simulink model "Factory"  (R2022b)
settings: Solver=VariableStepAuto  StartTime=0.0  StopTime=10.0  RelTol=1e-3
settings Model: Creator=Stefano  LastModifiedBy=stefanopanzieri
settings SolverCC: AlgebraicLoopSolver=TrustRegion
settings DebuggingCC: UnconnectedInputMsg=warning  UnconnectedOutputMsg=warning  UnconnectedLineMsg=warning  SFMachineParentedDataDiag=warning
settings ModelReferenceCC: EnableRefExpFcnMdlSchedulingChecks=on
settings SFSimCC: CustomCodeUndefinedFunction=UseInterfaceOnly
settings RTWCC: DLArmComputeVersion=19.05

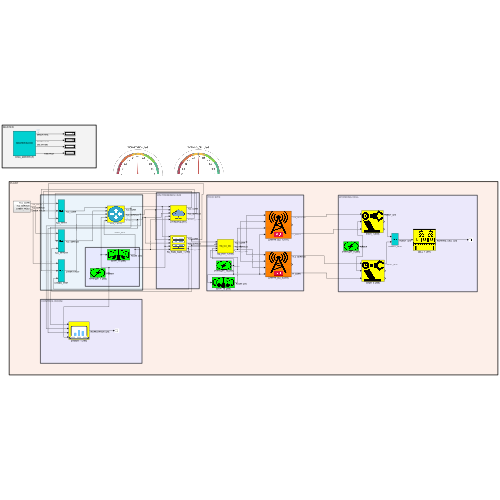
[thumbnail: Simulink's stored preview of the top-level diagram]
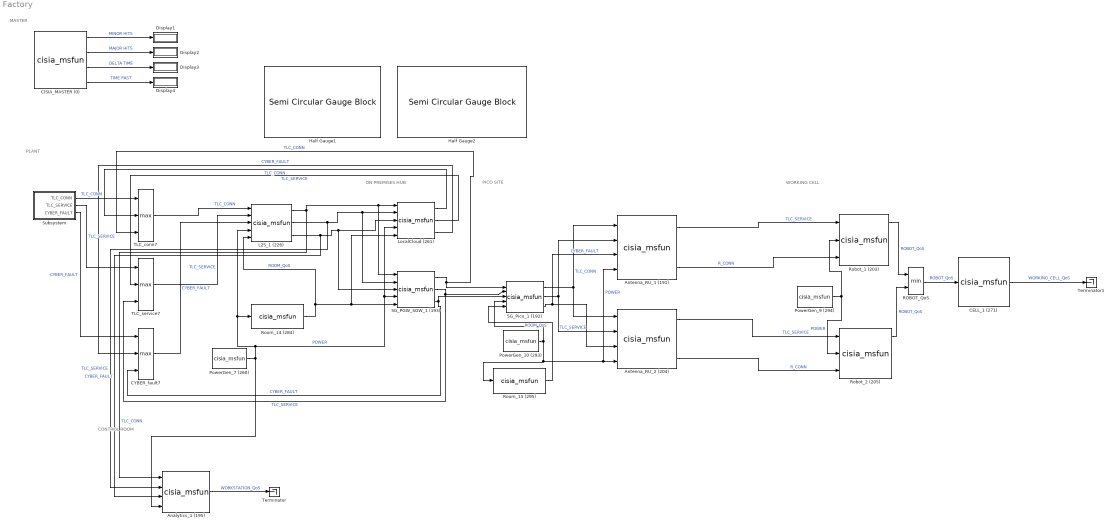
== system Factory ==
  note: WORKING CELL
  note: PICO SITE
  note: CONTROL ROOM
  note: ON PREMISES HUB
  note: PLANT
  note: MASTER
  5G_PGW_SGW_1 (193) : M-S-Function  FunctionName=cisia_msfun  Parameters=Parameter1, Parameter2, Parameter3, resources, Parameter10, codeupdate, step_received, step_computed, dynamic_computed, step_sended, id_entity, id_project, id_type, name_type, color  mask(S-function:msfcn_unit_delay){Parameter1='5G_PGW_SGW_1', Parameter2=1, Parameter3='ORO', resources=|, Parameter10=off, codeupdate=off, step_received=|, step_computed=, dynamic_computed=, step_sended=|, id_entity=193, id_project=34, id_type=40, name_type=App_Server, color=#00AAFF}
      mask resources=|
      | *** INPUT RESOURCES ***
      | NUM_INPUTS 5
      | TLC_CONN (20)
      | TLC_SERVICE (20)
      | CYBER_FAULT (10)
      | POWER (1)
      | ROOM_QoS (1)
      |
      | *** STATE VARIABLES ***
      | NUM_VARIABLES 24
      | Operative_Level(NUMERIC)(1)(1)
      | TLC_services(NUMERIC_ARRAY)(20)(0  0  0  0  0  0  0  0  0  0  0  0  0  0  0  0  0  0  0  0)
      | TLC_service_names(STRING)(100)()
      | Connection(NUMERIC_ARRAY)(20)(0  0  0  0  0  0  0  0  0  0  0  0  0  0  0  0  0  0  0  0)
      | Dos_attack(NUMERIC)(1)(0)
      | MITM_attack(NUMERIC)(1)(0)
      | Virus_Attack(NUMERIC)(1)(0)
      | Port_Scan_Attack(NUMERIC)(1)(0)
      | Cyber_Fault(NUMERIC_ARRAY)(10)(0  0  0  0  0  0  0  0  0  0)
      | BGP_hijacking(NUMERIC)(1)(0)
      | Mechanical_Fault(NUMERIC)(1)(0)
      | Cooling_Fault(NUMERIC)(1)(0)
      | Conn_Fault(NUMERIC)(1)(0)
      | Consumed_Services(NUMERIC_ARRAY)(20)(0  0  0  0  0  0  0  0  0  0  0  0  0  0  0  0  0  0  0  0)
      | Service_Fault(NUMERIC)(1)(0)
      | Redundancy_Fault(NUMERIC)(1)(0)
      | BotNet_Attack(NUMERIC)(1)(0)
      | Data_Corruption(NUMERIC)(1)(0)
      | syslog_adm_login(NUMERIC)(1)(0)
      | SW_Change(NUMERIC)(1)(0)
      | Config_Change(NUMERIC)(1)(0)
      | Port_Saturation(NUMERIC)(1)(0)
      | Congestion_Fault(NUMERIC)(1)(0)
      | TLC_revoke(NUMERIC_ARRAY)(20)(0  0  0  0  0  0  0  0  0  0  0  0  0  0  0  0  0  0  0  0)
      |
      | *** OUTPUT RESOURCES ***
      | NUM_OUTPUTS 3
      | TLC_CONN (20)
      | TLC_SERVICE (20)
      | CYBER_FAULT (10)
      mask step_received=|
      | Connection=max(Connection_init,TLC_CONN);
      | TLC_services=max(TLC_services_init,TLC_SERVICE);
      | TLC_services=mod(TLC_services,10);
      | TLC_revoke=floor(TLC_SERVICE/10);
      |
      | Mechanical_Fault=max([Mechanical_Fault Mechanical_Fault_init]);
      |
      | %if strcmp(name_entity,"BlockChainServer") && (cisia.major_time>=2)
      |  % Dos_attack=1;
      |  %TLC_revoke(9)=1;
      |  %TLC_services(9)=0;
      | %end
      |
      |
      | Cyber_Fault=max(CYBER_FAULT, transpose([Dos_attack   MITM_attack Virus_Attack Port_Scan_Attack  BGP_hijacking BotNet_Attack Data_Corruption SW_Change Config_Change Port_Saturation]));
      |
      | Service_Fault=max(abs(Consumed_Services.*TLC_services-Consumed_Services));
      | Redundancy_Fault=max(abs(Consumed_Services.*TLC_CONN-Consumed_Services));
      |
      | Conn_Fault=max([Dos_attack  Mechanical_Fault  1-POWER 1-ROOM_QoS] );
      |
      |
      | Operative_Level=(1-Conn_Fault)*(1-0.5*max(Cyber_Fault))*(1-Service_Fault)*max(max(TLC_CONN),0.5);
      mask step_sended=|
      | TLC_CONN=Connection*(1-Conn_Fault);
      | TLC_SERVICE=TLC_services*(1-Conn_Fault)*(1-Service_Fault)*(1-syslog_adm_login)+10*TLC_revoke;
      | CYBER_FAULT=Cyber_Fault*(1-Conn_Fault);
      mask prompts: Parameter1 "entity name"; Parameter2 "sampling time"; Parameter3 "project"; resources "input resources and state variables"; Parameter10 "Bring state variables to output"; codeupdate "update code from mask"
      mask help: This is a level-2 MATLAB file S-function which demonstrates CISIA entity
      mask DialogControl Container1 Prompt: All parameters
      mask Display: image('Icons/App_Server.png')
  5G_Pico_1 (192) : M-S-Function  FunctionName=cisia_msfun  Parameters=Parameter1, Parameter2, Parameter3, resources, Parameter10, codeupdate, step_received, step_computed, dynamic_computed, step_sended, id_entity, id_project, id_type, name_type, color  mask(S-function:msfcn_unit_delay){Parameter1='5G_Pico_1', Parameter2=1, Parameter3='ORO', resources=|, Parameter10=off, codeupdate=off, step_received=|, step_computed=, dynamic_computed=, step_sended=|, id_entity=192, id_project=34, id_type=42, name_type=5G_CU_DU, color=#FF00FF}
      mask resources=|
      | *** INPUT RESOURCES ***
      | NUM_INPUTS 5
      | TLC_CONN (20)
      | TLC_SERVICE (20)
      | CYBER_FAULT (10)
      | POWER (1)
      | ROOM_QoS (1)
      |
      | *** STATE VARIABLES ***
      | NUM_VARIABLES 20
      | Operative_Level(NUMERIC)(1)(1)
      | TLC_services(NUMERIC_ARRAY)(20)(0  0  0  0  0  0  0  0  0  0  0  0  0  0  0  0  0  0  0  0)
      | Connection(NUMERIC_ARRAY)(20)(0  0  0  0  0  0  0  0  0  0  0  0  0  0  0  0  0  0  0  0)
      | Dos_attack(NUMERIC)(1)(0)
      | MITM_attack(NUMERIC)(1)(0)
      | Virus_Attack(NUMERIC)(1)(0)
      | Port_Scan_Attack(NUMERIC)(1)(0)
      | Cyber_Fault(NUMERIC_ARRAY)(10)(0  0  0  0  0  0  0  0  0  0)
      | BGP_hijacking(NUMERIC)(1)(0)
      | Mechanical_Fault(NUMERIC)(1)(0)
      | Conn_Fault(NUMERIC)(1)(0)
      | Consumed_Services(NUMERIC_ARRAY)(20)(0  0  0  0  0  0  0  0  0  0  0  0  0  0  0  0  0  0  0  0)
      | Service_Fault(NUMERIC)(1)(0)
      | Redundancy_Fault(NUMERIC)(1)(0)
      | BotNet_Attack(NUMERIC)(1)(0)
      | Data_Corruption(NUMERIC)(1)(0)
      | SW_Change(NUMERIC)(1)(0)
      | Config_Change(NUMERIC)(1)(0)
      | Port_Saturation(NUMERIC)(1)(0)
      | TLC_revoke(NUMERIC_ARRAY)(20)(0  0  0  0  0  0  0  0  0  0  0  0  0  0  0  0  0  0  0  0)
      |
      | *** OUTPUT RESOURCES ***
      | NUM_OUTPUTS 3
      | TLC_CONN (20)
      | TLC_SERVICE (20)
      | CYBER_FAULT (10)
      mask step_received=|
      | Connection=max(Connection_init,TLC_CONN);
      | TLC_services=max(TLC_services_init,TLC_SERVICE);
      | TLC_services=mod(TLC_services,10);
      | TLC_revoke=floor(TLC_SERVICE/10);
      |
      | Cyber_Fault=max(CYBER_FAULT, transpose([Dos_attack   MITM_attack Virus_Attack Port_Scan_Attack  BGP_hijacking BotNet_Attack Data_Corruption SW_Change Config_Change Port_Saturation]));
      |
      | Conn_Fault=max([Dos_attack  Mechanical_Fault  1-POWER 1-ROOM_QoS] );
      |
      | Service_Fault=max(abs(Consumed_Services.*TLC_services-Consumed_Services));
      | Redundancy_Fault=max(abs(Consumed_Services.*TLC_CONN-Consumed_Services));
      |
      | Operative_Level=(1-Conn_Fault)*(1-0.5*max(Cyber_Fault))*(1-Service_Fault)*max(max(TLC_CONN),0.5);
      mask step_sended=|
      | TLC_CONN=Connection*(1-Conn_Fault);
      | TLC_SERVICE=TLC_services*(1-Conn_Fault)*(1-Service_Fault)+TLC_revoke*10;
      | CYBER_FAULT=Cyber_Fault*(1-Conn_Fault);
      mask prompts: Parameter1 "entity name"; Parameter2 "sampling time"; Parameter3 "project"; resources "input resources and state variables"; Parameter10 "Bring state variables to output"; codeupdate "update code from mask"
      mask help: This is a level-2 MATLAB file S-function which demonstrates CISIA entity
      mask DialogControl Container1 Prompt: All parameters
      mask Display: disp('5G_CU_DU')
  Analytics_1 (195) : M-S-Function  FunctionName=cisia_msfun  Parameters=Parameter1, Parameter2, Parameter3, resources, Parameter10, codeupdate, step_received, step_computed, dynamic_computed, step_sended, id_entity, id_project, id_type, name_type, color  mask(S-function:msfcn_unit_delay){Parameter1='Analytics_1', Parameter2=1, Parameter3='ORO', resources=|, Parameter10=off, codeupdate=off, step_received=|, step_computed=, dynamic_computed=, step_sended=WORKSTATION_QoS=Operative_Level;, id_entity=195, id_project=34, id_type=43, name_type=Workstation, color=#FFFFFF}
      mask resources=|
      | *** INPUT RESOURCES ***
      | NUM_INPUTS 4
      | TLC_CONN (20)
      | TLC_SERVICE (20)
      | CYBER_FAULT (10)
      | POWER (1)
      |
      | *** STATE VARIABLES ***
      | NUM_VARIABLES 18
      | Operative_Level(NUMERIC)(1)(1)
      | Connection(NUMERIC_ARRAY)(20)(0  0  0  0  0  0  0  0  0  0  0  0  0  0  0  0  0  0  0  0)
      | Dos_attack(NUMERIC)(1)(0)
      | MITM_attack(NUMERIC)(1)(0)
      | Virus_Attack(NUMERIC)(1)(0)
      | Port_Scan_Attack(NUMERIC)(1)(0)
      | Cyber_Fault(NUMERIC_ARRAY)(10)(0  0  0  0  0  0  0  0  0  0)
      | BGP_hijacking(NUMERIC)(1)(0)
      | Mechanical_Fault(NUMERIC)(1)(0)
      | Conn_Fault(NUMERIC)(1)(0)
      | Consumed_Services(NUMERIC_ARRAY)(20)(0  0  0  0  0  0  0  0  0  0  0  0  0  0  0  0  0  0  0  0)
      | Service_Fault(NUMERIC)(1)(0)
      | Redundancy_Fault(NUMERIC)(1)(0)
      | BotNet_Attack(NUMERIC)(1)(0)
      | Data_Corruption(NUMERIC)(1)(0)
      | SW_Change(NUMERIC)(1)(0)
      | Config_Change(NUMERIC)(1)(0)
      | Port_Saturation(NUMERIC)(1)(0)
      |
      | *** OUTPUT RESOURCES ***
      | NUM_OUTPUTS 1
      | WORKSTATION_QoS (1)
      mask step_received=|
      | Connection=max(Connection_init,TLC_CONN);
      |
      | Cyber_Fault=max(CYBER_FAULT, transpose([Dos_attack   MITM_attack Virus_Attack Port_Scan_Attack  BGP_hijacking BotNet_Attack Data_Corruption SW_Change Config_Change Port_Saturation]));
      |
      | % Vale 1 in presenza di fault
      | Conn_Fault=max([Dos_attack  Mechanical_Fault  1-POWER] );
      |
      |
      |
      | Operative_Level=(1-Conn_Fault)*max(max(TLC_CONN),0.5);
      mask prompts: Parameter1 "entity name"; Parameter2 "sampling time"; Parameter3 "project"; resources "input resources and state variables"; Parameter10 "Bring state variables to output"; codeupdate "update code from mask"
      mask help: This is a level-2 MATLAB file S-function which demonstrates CISIA entity
      mask DialogControl Container1 Prompt: All parameters
      mask Display: image('Icons/Analytics_1.png')
  Antenna_RU_1 (191) : M-S-Function  FunctionName=cisia_msfun  Parameters=Parameter1, Parameter2, Parameter3, resources, Parameter10, codeupdate, step_received, step_computed, dynamic_computed, step_sended, id_entity, id_project, id_type, name_type, color  mask(S-function:msfcn_unit_delay){Parameter1='Antenna_RU_1', Parameter2=1, Parameter3='ORO', resources=|, Parameter10=off, codeupdate=off, step_received=|, step_computed=, dynamic_computed=, step_sended=|, id_entity=191, id_project=34, id_type=41, name_type=RU_ANTENNA, color=#FFFFFF}
      mask resources=|
      | *** INPUT RESOURCES ***
      | NUM_INPUTS 4
      | TLC_CONN (20)
      | TLC_SERVICE (20)
      | CYBER_FAULT (10)
      | POWER (1)
      |
      | *** STATE VARIABLES ***
      | NUM_VARIABLES 24
      | Operative_Level(NUMERIC)(1)(1)
      | TLC_services(NUMERIC_ARRAY)(20)(0  0  0  0  0  0  0  0  0  0  0  0  0  0  0  0  0  0  0  0)
      | TLC_service_names(STRING)(100)()
      | Connection(NUMERIC_ARRAY)(20)(0  0  0  0  0  0  0  0  0  0  0  0  0  0  0  0  0  0  0  0)
      | Dos_attack(NUMERIC)(1)(0)
      | MITM_attack(NUMERIC)(1)(0)
      | Virus_Attack(NUMERIC)(1)(0)
      | Port_Scan_Attack(NUMERIC)(1)(0)
      | Cyber_Fault(NUMERIC_ARRAY)(10)(0  0  0  0  0  0  0  0  0  0)
      | BGP_hijacking(NUMERIC)(1)(0)
      | Mechanical_Fault(NUMERIC)(1)(0)
      | Power_Fault(NUMERIC)(1)(0)
      | Conn_Fault(NUMERIC)(1)(0)
      | Consumed_Services(NUMERIC_ARRAY)(20)(0  0  0  0  0  0  0  0  0  0  0  0  0  0  0  0  0  0  0  0)
      | Service_Fault(NUMERIC)(1)(0)
      | Redundancy_Fault(NUMERIC)(1)(0)
      | BotNet_Attack(NUMERIC)(1)(0)
      | Data_Corruption(NUMERIC)(1)(0)
      | SW_Change(NUMERIC)(1)(0)
      | Config_Change(NUMERIC)(1)(0)
      | Port_Saturation(NUMERIC)(1)(0)
      | Congestion_Fault(NUMERIC)(1)(0)
      | My_Service(NUMERIC)(1)(0)
      | TLC_revoke(NUMERIC_ARRAY)(20)(0  0  0  0  0  0  0  0  0  0  0  0  0  0  0  0  0  0  0  0)
      |
      | *** OUTPUT RESOURCES ***
      | NUM_OUTPUTS 3
      | TLC_SERVICE (20)
      | CYBER_FAULT (10)
      | R_CONN (20)
      mask step_received=|
      | Connection=max(Connection_init,TLC_CONN);
      | TLC_services=max(TLC_services_init,TLC_SERVICE);
      | TLC_services=mod(TLC_services,10);
      | TLC_revoke=floor(TLC_SERVICE/10);
      |
      | Cyber_Fault=max(CYBER_FAULT, transpose([Dos_attack   MITM_attack Virus_Attack Port_Scan_Attack  BGP_hijacking BotNet_Attack Data_Corruption SW_Change Config_Change Port_Saturation]));
      |
      | % Vale 1 in presenza di fault
      | Conn_Fault=max([Dos_attack  Mechanical_Fault  1-POWER] );
      |
      | Service_Fault=max(abs(Consumed_Services.*TLC_services-Consumed_Services));
      | Redundancy_Fault=max(abs(Consumed_Services.*TLC_CONN-Consumed_Services));
      |
      |
      | Operative_Level=(1-Conn_Fault)*max(max(TLC_services),0.5)*(1-Service_Fault)*(1-0.5*max(Cyber_Fault))*max(max(TLC_CONN),0.5);
      |
      | % Il servizio utilizzato
      | %My_Service=max([(1-Service_Fault) (1-Redundancy_Fault)/2]);
      mask step_sended=|
      | R_CONN=Connection*(1-Conn_Fault);
      | TLC_SERVICE=TLC_services*(1-Conn_Fault)+10*TLC_revoke;
      |
      | Cyber_Transmitted=min(Cyber_Fault, transpose([0 0 1 0 1 1 0 0 0 1]));
      | CYBER_FAULT=Cyber_Transmitted*(1-Conn_Fault);
      mask prompts: Parameter1 "entity name"; Parameter2 "sampling time"; Parameter3 "project"; resources "input resources and state variables"; Parameter10 "Bring state variables to output"; codeupdate "update code from mask"
      mask help: This is a level-2 MATLAB file S-function which demonstrates CISIA entity
      mask DialogControl Container1 Prompt: All parameters
      mask Display: image('Icons/RU_ANTENNA.png')
  Antenna_RU_2 (204) : M-S-Function  FunctionName=cisia_msfun  Parameters=Parameter1, Parameter2, Parameter3, resources, Parameter10, codeupdate, step_received, step_computed, dynamic_computed, step_sended, id_entity, id_project, id_type, name_type, color  mask(S-function:msfcn_unit_delay){Parameter1='Antenna_RU_2', Parameter2=1, Parameter3='ORO', resources=|, Parameter10=off, codeupdate=off, step_received=|, step_computed=, dynamic_computed=, step_sended=|, id_entity=204, id_project=34, id_type=41, name_type=RU_ANTENNA, color=#FFFFFF}
      mask resources=|
      | *** INPUT RESOURCES ***
      | NUM_INPUTS 4
      | TLC_CONN (20)
      | TLC_SERVICE (20)
      | CYBER_FAULT (10)
      | POWER (1)
      |
      | *** STATE VARIABLES ***
      | NUM_VARIABLES 24
      | Operative_Level(NUMERIC)(1)(1)
      | TLC_services(NUMERIC_ARRAY)(20)(0  0  0  0  0  0  0  0  0  0  0  0  0  0  0  0  0  0  0  0)
      | TLC_service_names(STRING)(100)()
      | Connection(NUMERIC_ARRAY)(20)(0  0  0  0  0  0  0  0  0  0  0  0  0  0  0  0  0  0  0  0)
      | Dos_attack(NUMERIC)(1)(0)
      | MITM_attack(NUMERIC)(1)(0)
      | Virus_Attack(NUMERIC)(1)(0)
      | Port_Scan_Attack(NUMERIC)(1)(0)
      | Cyber_Fault(NUMERIC_ARRAY)(10)(0  0  0  0  0  0  0  0  0  0)
      | BGP_hijacking(NUMERIC)(1)(0)
      | Mechanical_Fault(NUMERIC)(1)(0)
      | Power_Fault(NUMERIC)(1)(0)
      | Conn_Fault(NUMERIC)(1)(0)
      | Consumed_Services(NUMERIC_ARRAY)(20)(0  0  0  0  0  0  0  0  0  0  0  0  0  0  0  0  0  0  0  0)
      | Service_Fault(NUMERIC)(1)(0)
      | Redundancy_Fault(NUMERIC)(1)(0)
      | BotNet_Attack(NUMERIC)(1)(0)
      | Data_Corruption(NUMERIC)(1)(0)
      | SW_Change(NUMERIC)(1)(0)
      | Config_Change(NUMERIC)(1)(0)
      | Port_Saturation(NUMERIC)(1)(0)
      | Congestion_Fault(NUMERIC)(1)(0)
      | My_Service(NUMERIC)(1)(0)
      | TLC_revoke(NUMERIC_ARRAY)(20)(0  0  0  0  0  0  0  0  0  0  0  0  0  0  0  0  0  0  0  0)
      |
      | *** OUTPUT RESOURCES ***
      | NUM_OUTPUTS 3
      | TLC_SERVICE (20)
      | CYBER_FAULT (10)
      | R_CONN (20)
      mask step_received=|
      | Connection=max(Connection_init,TLC_CONN);
      | TLC_services=max(TLC_services_init,TLC_SERVICE);
      | TLC_services=mod(TLC_services,10);
      | TLC_revoke=floor(TLC_SERVICE/10);
      |
      | Cyber_Fault=max(CYBER_FAULT, transpose([Dos_attack   MITM_attack Virus_Attack Port_Scan_Attack  BGP_hijacking BotNet_Attack Data_Corruption SW_Change Config_Change Port_Saturation]));
      |
      | % Vale 1 in presenza di fault
      | Conn_Fault=max([Dos_attack  Mechanical_Fault  1-POWER] );
      |
      | Service_Fault=max(abs(Consumed_Services.*TLC_services-Consumed_Services));
      | Redundancy_Fault=max(abs(Consumed_Services.*TLC_CONN-Consumed_Services));
      |
      |
      | Operative_Level=(1-Conn_Fault)*max(max(TLC_services),0.5)*(1-Service_Fault)*(1-0.5*max(Cyber_Fault))*max(max(TLC_CONN),0.5);
      |
      | % Il servizio utilizzato
      | %My_Service=max([(1-Service_Fault) (1-Redundancy_Fault)/2]);
      mask step_sended=|
      | R_CONN=Connection*(1-Conn_Fault);
      | TLC_SERVICE=TLC_services*(1-Conn_Fault)+10*TLC_revoke;
      |
      | Cyber_Transmitted=min(Cyber_Fault, transpose([0 0 1 0 1 1 0 0 0 1]));
      | CYBER_FAULT=Cyber_Transmitted*(1-Conn_Fault);
      mask prompts: Parameter1 "entity name"; Parameter2 "sampling time"; Parameter3 "project"; resources "input resources and state variables"; Parameter10 "Bring state variables to output"; codeupdate "update code from mask"
      mask help: This is a level-2 MATLAB file S-function which demonstrates CISIA entity
      mask DialogControl Container1 Prompt: All parameters
      mask Display: image('Icons/RU_ANTENNA.png')
  CELL_1 (271) : M-S-Function  FunctionName=cisia_msfun  Parameters=Parameter1, Parameter2, Parameter3, resources, Parameter10, codeupdate, step_received, step_computed, dynamic_computed, step_sended, id_entity, id_project, id_type, name_type, color  mask(S-function:msfcn_unit_delay){Parameter1='CELL_1', Parameter2=1, Parameter3='ORO', resources=|, Parameter10=off, codeupdate=off, step_received=Operative_Level=ROBOT_QoS;, step_computed=, dynamic_computed=, step_sended=WORKING_CELL_QoS=Operative_Level;, id_entity=271, id_project=34, id_type=58, name_type=Working_Cell, color=#00FFAA}
      mask resources=|
      | *** INPUT RESOURCES ***
      | NUM_INPUTS 1
      | ROBOT_QoS (1)
      |
      | *** STATE VARIABLES ***
      | NUM_VARIABLES 1
      | Operative_Level(NUMERIC)(1)(1)
      |
      | *** OUTPUT RESOURCES ***
      | NUM_OUTPUTS 1
      | WORKING_CELL_QoS (1)
      mask prompts: Parameter1 "entity name"; Parameter2 "sampling time"; Parameter3 "project"; resources "input resources and state variables"; Parameter10 "Bring state variables to output"; codeupdate "update code from mask"
      mask help: This is a level-2 MATLAB file S-function which demonstrates CISIA entity
      mask DialogControl Container1 Prompt: All parameters
      mask Display: image('Icons/Working_Cell.png')
  CISIA_MASTER (0) : M-S-Function  FunctionName=cisia_msfun  Parameters=Parameter1, Parameter2, Parameter3, resources, Parameter4, Parameter5, Parameter6, Parameter7, Parameter8, Parameter9,Parameter11,Parameter12  mask(S-function:msfcn_unit_delay){Parameter1='CISIA_MASTER', Parameter2=[1], Parameter3='Factory', resources=off, Parameter4=on, Parameter5=off, Parameter6=off, Parameter7=off, Parameter8=0.001, Parameter9=off, Parameter11=on, Parameter12=off}
      mask prompts: Parameter1 "entity name"; Parameter2 "sampling time"; Parameter3 "project"; resources "Save status at each major hit"; Parameter4 "Show Operative Levels with colors"; Parameter5 "Load Entities from file"; Parameter6 "Load Start from Mask"; Parameter7 "Real Time"; Parameter8 "Real Time Hit (sec)"; Parameter9 "Skip saving"; Parameter11 "Show unconnected"; Parameter12 "Save port values"
      mask help:
      | MASTER BLOCK
      | v.2.0
      mask Display: disp('MASTER BLOCK')
  CYBER_fault7 : MinMax  Function=max  Inputs=3
  Display{1..4} (4 alike) : Display
  Half Gauge1 : SemiCircularGaugeBlock  ScaleMax=1
  Half Gauge2 : SemiCircularGaugeBlock  ScaleMax=1
  L2S_1 (226) : M-S-Function  FunctionName=cisia_msfun  Parameters=Parameter1, Parameter2, Parameter3, resources, Parameter10, codeupdate, step_received, step_computed, dynamic_computed, step_sended, id_entity, id_project, id_type, name_type, color  mask(S-function:msfcn_unit_delay){Parameter1='L2S_1', Parameter2=1, Parameter3='ORO', resources=|, Parameter10=off, codeupdate=off, step_received=|, step_computed=, dynamic_computed=, step_sended=|, id_entity=226, id_project=34, id_type=24, name_type=Layer2Switch, color=#FFFFFF}
      mask resources=|
      | *** INPUT RESOURCES ***
      | NUM_INPUTS 5
      | TLC_CONN (20)
      | TLC_SERVICE (20)
      | CYBER_FAULT (10)
      | POWER (1)
      | ROOM_QoS (1)
      |
      | *** STATE VARIABLES ***
      | NUM_VARIABLES 20
      | Operative_Level(NUMERIC)(1)(1)
      | TLC_services(NUMERIC_ARRAY)(20)(0  0  0  0  0  0  0  0  0  0  0  0  0  0  0  0  0  0  0  0)
      | TLC_service_names(STRING)(100)()
      | Connection(NUMERIC_ARRAY)(20)(0  0  0  0  0  0  0  0  0  0  0  0  0  0  0  0  0  0  0  0)
      | Dos_attack(NUMERIC)(1)(0)
      | MITM_attack(NUMERIC)(1)(0)
      | Virus_Attack(NUMERIC)(1)(0)
      | Port_Scan_Attack(NUMERIC)(1)(0)
      | Cyber_Fault(NUMERIC_ARRAY)(10)(0  0  0  0  0  0  0  0  0  0)
      | BGP_hijacking(NUMERIC)(1)(0)
      | Mechanical_Fault(NUMERIC)(1)(0)
      | Conn_Fault(NUMERIC)(1)(0)
      | Consumed_Services(NUMERIC_ARRAY)(20)(0  0  0  0  0  0  0  0  0  0  0  0  0  0  0  0  0  0  0  0)
      | Service_Fault(NUMERIC)(1)(0)
      | BotNet_Attack(NUMERIC)(1)(0)
      | Data_Corruption(NUMERIC)(1)(0)
      | SW_Change(NUMERIC)(1)(0)
      | Config_Change(NUMERIC)(1)(0)
      | Port_Saturation(NUMERIC)(1)(0)
      | TLC_revoke(NUMERIC_ARRAY)(20)(0  0  0  0  0  0  0  0  0  0  0  0  0  0  0  0  0  0  0  0)
      |
      | *** OUTPUT RESOURCES ***
      | NUM_OUTPUTS 3
      | TLC_CONN (20)
      | TLC_SERVICE (20)
      | CYBER_FAULT (10)
      mask step_received=|
      | Connection=max(Connection_init,TLC_CONN);
      | TLC_services=max(TLC_services_init,TLC_SERVICE);
      | TLC_services=mod(TLC_services,10);
      | TLC_revoke=floor(TLC_SERVICE/10);
      |
      | Cyber_Fault=max(CYBER_FAULT, transpose([Dos_attack   MITM_attack Virus_Attack Port_Scan_Attack  BGP_hijacking BotNet_Attack Data_Corruption SW_Change Config_Change Port_Saturation]));
      |
      | Conn_Fault=max([Dos_attack  Mechanical_Fault  1-POWER 1-ROOM_QoS] );
      |
      | Service_Fault=max(abs(Consumed_Services.*TLC_services-Consumed_Services));
      | Redundancy_Fault=max(abs(Consumed_Services.*TLC_CONN-Consumed_Services));
      |
      | Operative_Level=(1-Conn_Fault)*(1-0.5*max(Cyber_Fault))*(1-Service_Fault)*max(max(TLC_CONN),0.5);
      mask step_sended=|
      | TLC_CONN=Connection*(1-Conn_Fault);
      | TLC_SERVICE=TLC_services*(1-Conn_Fault)*(1-Service_Fault)+10*TLC_revoke;
      |
      | Cyber_Transmitted=min(Cyber_Fault, transpose([0 0 1 0 1 1 0 0 0 1]));
      | CYBER_FAULT=Cyber_Transmitted*(1-Conn_Fault);
      mask prompts: Parameter1 "entity name"; Parameter2 "sampling time"; Parameter3 "project"; resources "input resources and state variables"; Parameter10 "Bring state variables to output"; codeupdate "update code from mask"
      mask help: This is a level-2 MATLAB file S-function which demonstrates CISIA entity
      mask DialogControl Container1 Prompt: All parameters
      mask Display: image('Icons/Layer2Switch.png')
  LocalCloud (261) : M-S-Function  FunctionName=cisia_msfun  Parameters=Parameter1, Parameter2, Parameter3, resources, Parameter10, codeupdate, step_received, step_computed, dynamic_computed, step_sended, id_entity, id_project, id_type, name_type, color  mask(S-function:msfcn_unit_delay){Parameter1='LocalCloud', Parameter2=1, Parameter3='ORO', resources=|, Parameter10=off, codeupdate=off, step_received=|, step_computed=, dynamic_computed=, step_sended=|, id_entity=261, id_project=34, id_type=53, name_type=CloudServer, color=#FFFFFF}
      mask resources=|
      | *** INPUT RESOURCES ***
      | NUM_INPUTS 5
      | TLC_CONN (20)
      | TLC_SERVICE (20)
      | CYBER_FAULT (10)
      | POWER (1)
      | ROOM_QoS (1)
      |
      | *** STATE VARIABLES ***
      | NUM_VARIABLES 20
      | Operative_Level(NUMERIC)(1)(1)
      | TLC_services(NUMERIC_ARRAY)(20)(0  0  0  0  0  0  0  0  0  0  0  0  0  0  0  0  0  0  0  0)
      | Connection(NUMERIC_ARRAY)(20)(0  0  0  0  0  0  0  0  0  0  0  0  0  0  0  0  0  0  0  0)
      | Dos_attack(NUMERIC)(1)(0)
      | MITM_attack(NUMERIC)(1)(0)
      | Virus_Attack(NUMERIC)(1)(0)
      | Port_Scan_Attack(NUMERIC)(1)(0)
      | Cyber_Fault(NUMERIC_ARRAY)(10)(0  0  0  0  0  0  0  0  0  0)
      | BGP_hijacking(NUMERIC)(1)(0)
      | Mechanical_Fault(NUMERIC)(1)(0)
      | Conn_Fault(NUMERIC)(1)(0)
      | Consumed_Services(NUMERIC_ARRAY)(20)(0  0  0  0  0  0  0  0  0  0  0  0  0  0  0  0  0  0  0  0)
      | Service_Fault(NUMERIC)(1)(0)
      | Redundancy_Fault(NUMERIC)(1)(0)
      | BotNet_Attack(NUMERIC)(1)(0)
      | Data_Corruption(NUMERIC)(1)(0)
      | SW_Change(NUMERIC)(1)(0)
      | Config_Change(NUMERIC)(1)(0)
      | Port_Saturation(NUMERIC)(1)(0)
      | TLC_revoke(NUMERIC_ARRAY)(20)(0  0  0  0  0  0  0  0  0  0  0  0  0  0  0  0  0  0  0  0)
      |
      | *** OUTPUT RESOURCES ***
      | NUM_OUTPUTS 3
      | TLC_CONN (20)
      | TLC_SERVICE (20)
      | CYBER_FAULT (10)
      mask step_received=|
      | Connection=max(Connection_init,TLC_CONN);
      | TLC_services=max(TLC_services_init,TLC_SERVICE);
      | TLC_services=mod(TLC_services,10);
      | TLC_revoke=floor(TLC_SERVICE/10);
      |
      | %TLC_services=max(TLC_services_init*(1+cisia.major_time),TLC_SERVICE);
      |
      |
      | Mechanical_Fault=max([Mechanical_Fault Mechanical_Fault_init]);
      |
      | Cyber_Fault=max(CYBER_FAULT, transpose([Dos_attack   MITM_attack Virus_Attack Port_Scan_Attack  BGP_hijacking BotNet_Attack Data_Corruption SW_Change Config_Change Port_Saturation]));
      |
      | Conn_Fault=max([Dos_attack  Mechanical_Fault  1-POWER 1-ROOM_QoS] );
      |
      | Service_Fault=max(abs(Consumed_Services.*TLC_services-Consumed_Services));
      | Redundancy_Fault=max(abs(Consumed_Services.*TLC_CONN-Consumed_Services));
      |
      | Operative_Level=(1-Conn_Fault)*(1-0.5*max(Cyber_Fault))*(1-Service_Fault)*max(max(TLC_CONN),0.5);
      mask step_sended=|
      | TLC_CONN=Connection*(1-Conn_Fault);
      | TLC_SERVICE=TLC_services*(1-Conn_Fault)*(1-Service_Fault)+10*TLC_revoke;
      | CYBER_FAULT=Cyber_Fault*(1-Conn_Fault);
      mask prompts: Parameter1 "entity name"; Parameter2 "sampling time"; Parameter3 "project"; resources "input resources and state variables"; Parameter10 "Bring state variables to output"; codeupdate "update code from mask"
      mask help: This is a level-2 MATLAB file S-function which demonstrates CISIA entity
      mask DialogControl Container1 Prompt: All parameters
      mask Display: image('Icons/CloudServer.png')
  PowerGen_10 (293) : M-S-Function  FunctionName=cisia_msfun  Parameters=Parameter1, Parameter2, Parameter3, resources, Parameter10, codeupdate, step_received, step_computed, dynamic_computed, step_sended, id_entity, id_project, id_type, name_type, color  mask(S-function:msfcn_unit_delay){Parameter1='PowerGen_10', Parameter2=1, Parameter3='ORO', resources=|, Parameter10=off, codeupdate=off, step_received=Operative_Level=1-Power_Fault;, step_computed=, dynamic_computed=, step_sended=POWER=Operative_Level;, id_entity=293, id_project=34, id_type=8, name_type=PowerSource, color=#84BD8C}
      mask resources=|
      | *** INPUT RESOURCES ***
      | NUM_INPUTS 0
      |
      | *** STATE VARIABLES ***
      | NUM_VARIABLES 2
      | Operative_Level(NUMERIC)(1)(1)
      | Power_Fault(NUMERIC)(1)(0)
      |
      | *** OUTPUT RESOURCES ***
      | NUM_OUTPUTS 1
      | POWER (1)
      mask prompts: Parameter1 "entity name"; Parameter2 "sampling time"; Parameter3 "project"; resources "input resources and state variables"; Parameter10 "Bring state variables to output"; codeupdate "update code from mask"
      mask help: This is a level-2 MATLAB file S-function which demonstrates CISIA entity
      mask DialogControl Container1 Prompt: All parameters
      mask Display: image('Icons/PowerSource.png')
  PowerGen_7 (260) : M-S-Function  FunctionName=cisia_msfun  Parameters=Parameter1, Parameter2, Parameter3, resources, Parameter10, codeupdate, step_received, step_computed, dynamic_computed, step_sended, id_entity, id_project, id_type, name_type, color  mask(S-function:msfcn_unit_delay){Parameter1='PowerGen_7', Parameter2=1, Parameter3='ORO', resources=|, Parameter10=off, codeupdate=off, step_received=Operative_Level=1-Power_Fault;, step_computed=, dynamic_computed=, step_sended=POWER=Operative_Level;, id_entity=260, id_project=34, id_type=8, name_type=PowerSource, color=#84BD8C}
      mask resources=|
      | *** INPUT RESOURCES ***
      | NUM_INPUTS 0
      |
      | *** STATE VARIABLES ***
      | NUM_VARIABLES 2
      | Operative_Level(NUMERIC)(1)(1)
      | Power_Fault(NUMERIC)(1)(0)
      |
      | *** OUTPUT RESOURCES ***
      | NUM_OUTPUTS 1
      | POWER (1)
      mask prompts: Parameter1 "entity name"; Parameter2 "sampling time"; Parameter3 "project"; resources "input resources and state variables"; Parameter10 "Bring state variables to output"; codeupdate "update code from mask"
      mask help: This is a level-2 MATLAB file S-function which demonstrates CISIA entity
      mask DialogControl Container1 Prompt: All parameters
      mask Display: image('Icons/PowerSource.png')
  PowerGen_9 (294) : M-S-Function  FunctionName=cisia_msfun  Parameters=Parameter1, Parameter2, Parameter3, resources, Parameter10, codeupdate, step_received, step_computed, dynamic_computed, step_sended, id_entity, id_project, id_type, name_type, color  mask(S-function:msfcn_unit_delay){Parameter1='PowerGen_9', Parameter2=1, Parameter3='ORO', resources=|, Parameter10=off, codeupdate=off, step_received=Operative_Level=1-Power_Fault;, step_computed=, dynamic_computed=, step_sended=POWER=Operative_Level;, id_entity=294, id_project=34, id_type=8, name_type=PowerSource, color=#84BD8C}
      mask resources=|
      | *** INPUT RESOURCES ***
      | NUM_INPUTS 0
      |
      | *** STATE VARIABLES ***
      | NUM_VARIABLES 2
      | Operative_Level(NUMERIC)(1)(1)
      | Power_Fault(NUMERIC)(1)(0)
      |
      | *** OUTPUT RESOURCES ***
      | NUM_OUTPUTS 1
      | POWER (1)
      mask prompts: Parameter1 "entity name"; Parameter2 "sampling time"; Parameter3 "project"; resources "input resources and state variables"; Parameter10 "Bring state variables to output"; codeupdate "update code from mask"
      mask help: This is a level-2 MATLAB file S-function which demonstrates CISIA entity
      mask DialogControl Container1 Prompt: All parameters
      mask Display: image('Icons/PowerSource.png')
  ROBOT_QoS : MinMax  Inputs=2
  Robot_1 (203) : M-S-Function  FunctionName=cisia_msfun  Parameters=Parameter1, Parameter2, Parameter3, resources, Parameter10, codeupdate, step_received, step_computed, dynamic_computed, step_sended, id_entity, id_project, id_type, name_type, color  mask(S-function:msfcn_unit_delay){Parameter1='Robot_1', Parameter2=1, Parameter3='ORO', resources=|, Parameter10=off, codeupdate=off, step_received=|, step_computed=, dynamic_computed=, step_sended=|, id_entity=203, id_project=34, id_type=44, name_type=Robot, color=#FFFFFF}
      mask resources=|
      | *** INPUT RESOURCES ***
      | NUM_INPUTS 3
      | TLC_SERVICE (20)
      | POWER (1)
      | R_CONN (20)
      |
      | *** STATE VARIABLES ***
      | NUM_VARIABLES 12
      | Operative_Level(NUMERIC)(1)(1)
      | TLC_services(NUMERIC_ARRAY)(20)(0  0  0  0  0  0  0  0  0  0  0  0  0  0  0  0  0  0  0  0)
      | Connection(NUMERIC_ARRAY)(20)(0  0  0  0  0  0  0  0  0  0  0  0  0  0  0  0  0  0  0  0)
      | Mechanical_Fault(NUMERIC)(1)(0)
      | Consumed_Services(NUMERIC_ARRAY)(20)(0  0  0  0  0  0  0  0  0  0  0  0  0  0  0  0  0  0  0  0)
      | Service_Fault(NUMERIC)(1)(0)
      | Redundancy_Fault(NUMERIC)(1)(0)
      | Physical_Fault(NUMERIC)(1)(0)
      | TLC_revoke(NUMERIC_ARRAY)(20)(0  0  0  0  0  0  0  0  0  0  0  0  0  0  0  0  0  0  0  0)
      | Alternative_Services(NUMERIC_ARRAY)(20)(0  0  0  0  0  0  0  0  0  0  0  0  0  0  0  0  0  0  0  0)
      | Alt_Serv_Fault(NUMERIC)(1)(0)
      | Alt_Rout_Fault(NUMERIC)(1)(0)
      |
      | *** OUTPUT RESOURCES ***
      | NUM_OUTPUTS 3
      | ROBOT_QoS (1)
      | ALT_ROUTING (1)
      | ALT_SERVICES (1)
      mask step_received=|
      | Connection=max(Connection_init,R_CONN);
      | TLC_services=max(TLC_services_init,TLC_SERVICE);
      | TLC_services=mod(TLC_services,10);
      | TLC_revoke=floor(TLC_SERVICE/10);
      |
      | Physical_Fault=max([Mechanical_Fault  1-POWER] );
      |
      | Service_Fault=max(abs(Consumed_Services.*TLC_services-Consumed_Services));
      | Redundancy_Fault=max(abs(Consumed_Services.*R_CONN-Consumed_Services));
      |
      |
      | Alt_Serv_Fault=max(abs(Alternative_Services.*R_CONN-Alternative_Services));
      |
      | Alt_Rout_Fault=max(abs(Consumed_Services.*R_CONN-Consumed_Services));
      |
      |
      | Operative_Level=(1-Physical_Fault)*max(max(R_CONN),0.5)*(1-0.6*Service_Fault);
      mask step_sended=|
      | ROBOT_QoS=Operative_Level;
      |
      |
      | ALT_SERVICES=1-Alt_Serv_Fault;
      | ALT_ROUTING=1-Alt_Rout_Fault;
      mask prompts: Parameter1 "entity name"; Parameter2 "sampling time"; Parameter3 "project"; resources "input resources and state variables"; Parameter10 "Bring state variables to output"; codeupdate "update code from mask"
      mask help: This is a level-2 MATLAB file S-function which demonstrates CISIA entity
      mask DialogControl Container1 Prompt: All parameters
      mask Display: image('Icons/Robot.png')
  Robot_2 (205) : M-S-Function  FunctionName=cisia_msfun  Parameters=Parameter1, Parameter2, Parameter3, resources, Parameter10, codeupdate, step_received, step_computed, dynamic_computed, step_sended, id_entity, id_project, id_type, name_type, color  mask(S-function:msfcn_unit_delay){Parameter1='Robot_2', Parameter2=1, Parameter3='ORO', resources=|, Parameter10=off, codeupdate=off, step_received=|, step_computed=, dynamic_computed=, step_sended=|, id_entity=205, id_project=34, id_type=44, name_type=Robot, color=#FFFFFF}
      mask resources=|
      | *** INPUT RESOURCES ***
      | NUM_INPUTS 3
      | TLC_SERVICE (20)
      | POWER (1)
      | R_CONN (20)
      |
      | *** STATE VARIABLES ***
      | NUM_VARIABLES 12
      | Operative_Level(NUMERIC)(1)(1)
      | TLC_services(NUMERIC_ARRAY)(20)(0  0  0  0  0  0  0  0  0  0  0  0  0  0  0  0  0  0  0  0)
      | Connection(NUMERIC_ARRAY)(20)(0  0  0  0  0  0  0  0  0  0  0  0  0  0  0  0  0  0  0  0)
      | Mechanical_Fault(NUMERIC)(1)(0)
      | Consumed_Services(NUMERIC_ARRAY)(20)(0  0  0  0  0  0  0  0  0  0  0  0  0  0  0  0  0  0  0  0)
      | Service_Fault(NUMERIC)(1)(0)
      | Redundancy_Fault(NUMERIC)(1)(0)
      | Physical_Fault(NUMERIC)(1)(0)
      | TLC_revoke(NUMERIC_ARRAY)(20)(0  0  0  0  0  0  0  0  0  0  0  0  0  0  0  0  0  0  0  0)
      | Alternative_Services(NUMERIC_ARRAY)(20)(0  0  0  0  0  0  0  0  0  0  0  0  0  0  0  0  0  0  0  0)
      | Alt_Serv_Fault(NUMERIC)(1)(0)
      | Alt_Rout_Fault(NUMERIC)(1)(0)
      |
      | *** OUTPUT RESOURCES ***
      | NUM_OUTPUTS 3
      | ROBOT_QoS (1)
      | ALT_ROUTING (1)
      | ALT_SERVICES (1)
      mask step_received=|
      | Connection=max(Connection_init,R_CONN);
      | TLC_services=max(TLC_services_init,TLC_SERVICE);
      | TLC_services=mod(TLC_services,10);
      | TLC_revoke=floor(TLC_SERVICE/10);
      |
      | Physical_Fault=max([Mechanical_Fault  1-POWER] );
      |
      | Service_Fault=max(abs(Consumed_Services.*TLC_services-Consumed_Services));
      | Redundancy_Fault=max(abs(Consumed_Services.*R_CONN-Consumed_Services));
      |
      |
      | Alt_Serv_Fault=max(abs(Alternative_Services.*R_CONN-Alternative_Services));
      |
      | Alt_Rout_Fault=max(abs(Consumed_Services.*R_CONN-Consumed_Services));
      |
      |
      | Operative_Level=(1-Physical_Fault)*max(max(R_CONN),0.5)*(1-0.6*Service_Fault);
      mask step_sended=|
      | ROBOT_QoS=Operative_Level;
      |
      |
      | ALT_SERVICES=1-Alt_Serv_Fault;
      | ALT_ROUTING=1-Alt_Rout_Fault;
      mask prompts: Parameter1 "entity name"; Parameter2 "sampling time"; Parameter3 "project"; resources "input resources and state variables"; Parameter10 "Bring state variables to output"; codeupdate "update code from mask"
      mask help: This is a level-2 MATLAB file S-function which demonstrates CISIA entity
      mask DialogControl Container1 Prompt: All parameters
      mask Display: image('Icons/Robot.png')
  Room_14 (284) : M-S-Function  FunctionName=cisia_msfun  Parameters=Parameter1, Parameter2, Parameter3, resources, Parameter10, codeupdate, step_received, step_computed, dynamic_computed, step_sended, id_entity, id_project, id_type, name_type, color  mask(S-function:msfcn_unit_delay){Parameter1='Room_14', Parameter2=1, Parameter3='ORO', resources=|, Parameter10=off, codeupdate=off, step_received=|, step_computed=, dynamic_computed=, step_sended=ROOM_QoS=Operative_Level;, id_entity=284, id_project=34, id_type=9, name_type=Room, color=#EDB120}
      mask resources=|
      | *** INPUT RESOURCES ***
      | NUM_INPUTS 1
      | POWER (1)
      |
      | *** STATE VARIABLES ***
      | NUM_VARIABLES 8
      | Operative_Level(NUMERIC)(1)(1)
      | Power_Fault(NUMERIC)(1)(0)
      | Cooling_Fault(NUMERIC)(1)(0)
      | Flooding_Fault(NUMERIC)(1)(0)
      | Fire_Fault(NUMERIC)(1)(0)
      | Unauthorized_Access(NUMERIC)(1)(0)
      | Earthquake_Fault(NUMERIC)(1)(0)
      | Physical_Fault(NUMERIC)(1)(0)
      |
      | *** OUTPUT RESOURCES ***
      | NUM_OUTPUTS 1
      | ROOM_QoS (1)
      mask step_received=|
      | Physical_Fault=max([Power_Fault Flooding_Fault Fire_Fault Cooling_Fault 1-POWER]);
      |
      |
      | %Operative_Level=min([1-Power_Fault 1-Flooding_Fault  1-Fire_Fault  1-Cooling_Fault  POWER]);
      | %Operative_Level=Operative_Level*max((1-Unauthorized_Access),0.5);
      |
      | Operative_Level=(1-Physical_Fault)*(1-0.5*Unauthorized_Access);
      mask prompts: Parameter1 "entity name"; Parameter2 "sampling time"; Parameter3 "project"; resources "input resources and state variables"; Parameter10 "Bring state variables to output"; codeupdate "update code from mask"
      mask help: This is a level-2 MATLAB file S-function which demonstrates CISIA entity
      mask DialogControl Container1 Prompt: All parameters
      mask Display: image('Icons/Room.png')
  Room_15 (295) : M-S-Function  FunctionName=cisia_msfun  Parameters=Parameter1, Parameter2, Parameter3, resources, Parameter10, codeupdate, step_received, step_computed, dynamic_computed, step_sended, id_entity, id_project, id_type, name_type, color  mask(S-function:msfcn_unit_delay){Parameter1='Room_15', Parameter2=1, Parameter3='ORO', resources=|, Parameter10=off, codeupdate=off, step_received=|, step_computed=, dynamic_computed=, step_sended=ROOM_QoS=Operative_Level;, id_entity=295, id_project=34, id_type=9, name_type=Room, color=#EDB120}
      mask resources=|
      | *** INPUT RESOURCES ***
      | NUM_INPUTS 1
      | POWER (1)
      |
      | *** STATE VARIABLES ***
      | NUM_VARIABLES 8
      | Operative_Level(NUMERIC)(1)(1)
      | Power_Fault(NUMERIC)(1)(0)
      | Cooling_Fault(NUMERIC)(1)(0)
      | Flooding_Fault(NUMERIC)(1)(0)
      | Fire_Fault(NUMERIC)(1)(0)
      | Unauthorized_Access(NUMERIC)(1)(0)
      | Earthquake_Fault(NUMERIC)(1)(0)
      | Physical_Fault(NUMERIC)(1)(0)
      |
      | *** OUTPUT RESOURCES ***
      | NUM_OUTPUTS 1
      | ROOM_QoS (1)
      mask step_received=|
      | Physical_Fault=max([Power_Fault Flooding_Fault Fire_Fault Cooling_Fault 1-POWER]);
      |
      |
      | %Operative_Level=min([1-Power_Fault 1-Flooding_Fault  1-Fire_Fault  1-Cooling_Fault  POWER]);
      | %Operative_Level=Operative_Level*max((1-Unauthorized_Access),0.5);
      |
      | Operative_Level=(1-Physical_Fault)*(1-0.5*Unauthorized_Access);
      mask prompts: Parameter1 "entity name"; Parameter2 "sampling time"; Parameter3 "project"; resources "input resources and state variables"; Parameter10 "Bring state variables to output"; codeupdate "update code from mask"
      mask help: This is a level-2 MATLAB file S-function which demonstrates CISIA entity
      mask DialogControl Container1 Prompt: All parameters
      mask Display: image('Icons/Room.png')
  Subsystem : Subsystem
  TLC_conn7 : MinMax  Function=max  Inputs=3
  TLC_service7 : MinMax  Function=max  Inputs=3
  Terminator : Terminator
  Terminator1 : Terminator
  wires:
  PowerGen_7 (260)/1 -> Analytics_1 (195)/4, LocalCloud (261)/4, 5G_PGW_SGW_1 (193)/4, Room_14 (284)/1, L2S_1 (226)/4  "POWER"
  Room_14 (284)/1 -> LocalCloud (261)/5, 5G_PGW_SGW_1 (193)/5, L2S_1 (226)/5  "ROOM_QoS"
  TLC_conn7/1 -> L2S_1 (226)/1  "TLC_CONN"
  TLC_service7/1 -> L2S_1 (226)/2  "TLC_SERVICE"
  CYBER_fault7/1 -> L2S_1 (226)/3  "CYBER_FAULT"
  LocalCloud (261)/1 -> TLC_conn7/2  "TLC_CONN"
  LocalCloud (261)/2 -> TLC_service7/2  "TLC_SERVICE"
  LocalCloud (261)/3 -> CYBER_fault7/2  "CYBER_FAULT"
  5G_PGW_SGW_1 (193)/1 -> 5G_Pico_1 (192)/1, TLC_conn7/3  "TLC_CONN"
  5G_PGW_SGW_1 (193)/2 -> 5G_Pico_1 (192)/2, TLC_service7/3  "TLC_SERVICE"
  5G_PGW_SGW_1 (193)/3 -> CYBER_fault7/3, 5G_Pico_1 (192)/3  "CYBER_FAULT"
  L2S_1 (226)/1 -> Analytics_1 (195)/1, 5G_PGW_SGW_1 (193)/1, LocalCloud (261)/1  "TLC_CONN"
  L2S_1 (226)/2 -> Analytics_1 (195)/2, 5G_PGW_SGW_1 (193)/2, LocalCloud (261)/2  "TLC_SERVICE"
  L2S_1 (226)/3 -> Analytics_1 (195)/3, 5G_PGW_SGW_1 (193)/3, LocalCloud (261)/3  "CYBER_FAULT"
  5G_Pico_1 (192)/1 -> Antenna_RU_2 (204)/1, Antenna_RU_1 (191)/1  "TLC_CONN"
  5G_Pico_1 (192)/2 -> Antenna_RU_2 (204)/2, Antenna_RU_1 (191)/2  "TLC_SERVICE"
  5G_Pico_1 (192)/3 -> Antenna_RU_2 (204)/3, Antenna_RU_1 (191)/3  "CYBER_FAULT"
  Robot_1 (203)/1 -> ROBOT_QoS/1  "ROBOT_QoS"
  ROBOT_QoS/1 -> CELL_1 (271)/1  "ROBOT_QoS"
  Robot_2 (205)/1 -> ROBOT_QoS/2  "ROBOT_QoS"
  PowerGen_10 (293)/1 -> Room_15 (295)/1, Antenna_RU_1 (191)/4, Antenna_RU_2 (204)/4, 5G_Pico_1 (192)/4  "POWER"
  Subsystem/1(TLC_CONN) -> TLC_conn7/1  "TLC_CONN"
  Subsystem/2(TLC_SERVICE) -> TLC_service7/1  "TLC_SERVICE"
  Subsystem/3(CYBER_FAULT) -> CYBER_fault7/1  "CYBER_FAULT"
  Room_15 (295)/1 -> 5G_Pico_1 (192)/5  "ROOM_QoS"
  Antenna_RU_1 (191)/3 -> Robot_1 (203)/3  "R_CONN"
  Antenna_RU_2 (204)/3 -> Robot_2 (205)/3  "R_CONN"
  PowerGen_9 (294)/1 -> Robot_1 (203)/2, Robot_2 (205)/2  "POWER"
  Antenna_RU_1 (191)/1 -> Robot_1 (203)/1  "TLC_SERVICE"
  Antenna_RU_2 (204)/1 -> Robot_2 (205)/1  "TLC_SERVICE"
  CISIA_MASTER (0)/4 -> Display4/1  "TIME PAST"
  CISIA_MASTER (0)/3 -> Display3/1  "DELTA TIME"
  CISIA_MASTER (0)/2 -> Display2/1  "MAJOR HITS"
  CISIA_MASTER (0)/1 -> Display1/1  "MINOR HITS"
  Analytics_1 (195)/1 -> Terminator/1  "WORKSTATION_QoS"
  CELL_1 (271)/1 -> Terminator1/1  "WORKING_CELL_QoS"

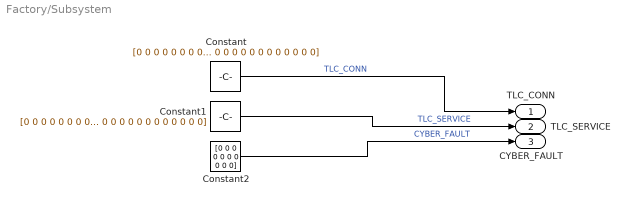
== system Factory/Subsystem ==
  Constant : Constant  Value=[0 0 0 0 0 0 0 0 0 0 0 0 0 0 0 0 0 0 0 0]
  Constant1 : Constant  Value=[0 0 0 0 0 0 0 0 0 0 0 0 0 0 0 0 0 0 0 0]
  Constant2 : Constant  Value=[0 0 0 0 0 0 0 0 0 0]
  TLC_CONN : Outport
  TLC_SERVICE : Outport  Port=2
  CYBER_FAULT : Outport  Port=3
  wires:
  Constant2/1 -> CYBER_FAULT/1  "CYBER_FAULT"
  Constant/1 -> TLC_CONN/1  "TLC_CONN"
  Constant1/1 -> TLC_SERVICE/1  "TLC_SERVICE"
